simulink model "plcTest"  (R2018a)
settings: Solver=VariableStepAuto  StartTime=0.0  StopTime=5  RelTol=1e-3
values from neighbouring files (symbols this model uses):
  structureType = -1.0    [test.sldd]
undefined symbols (not defined in the file or in its folder): a_elem, b_elem, DB1
libraries: plcLibrary x1
settings Model: DataDictionary=test.sldd  Creator=thomas  LastModifiedBy=thomas

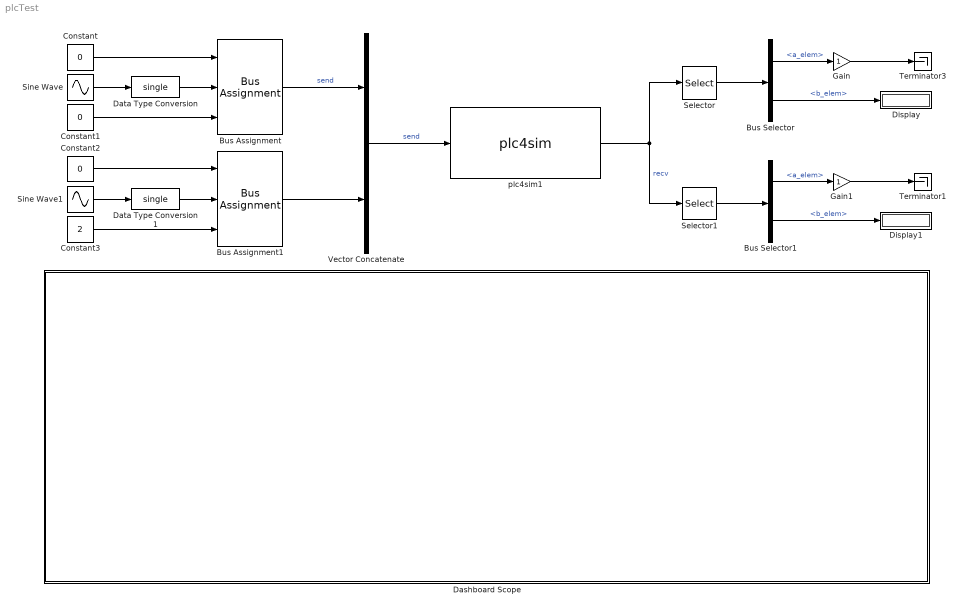
== system plcTest ==
  Bus Assignment : BusAssignment  AssignedSignals=a_elem,b_elem
  Bus Assignment1 : BusAssignment  AssignedSignals=a_elem,b_elem
  Bus Selector : BusSelector  OutputSignals=a_elem,b_elem
  Bus Selector1 : BusSelector  OutputSignals=a_elem,b_elem
  Constant : Constant  Value=0  OutDataTypeStr=Bus: structureType
  Constant1 : Constant  Value=0  OutDataTypeStr=uint8
  Constant2 : Constant  Value=0  OutDataTypeStr=Bus: structureType
  Constant3 : Constant  Value=2  OutDataTypeStr=uint8
  Dashboard Scope : Subsystem  DialogController=hmiCreateDDGDialog  IsWebBlock=on  mask(MWDashboardBlock){webBlockId=307e5b85-c1be-4a92-a345-0b0d646f5c8b, webBlockType=sdiscope, ShowInitialText=on, HMISrcModelName=plcTest}
      mask prompts: webBlockId "WebBlock Id"; webBlockType "WebBlock Type"; HMISrcModelName "Source Model"
      mask help: SimulinkHMI:dialogs:HMIScopeDialogDesc
      mask Help: helpview([docroot '/mapfiles/simulink.map'], 'hmi_scope')
      mask Display:
      | if strcmp(get_param(bdroot(gcb),'BlockDiagramType'), 'library')
      |     image([(matlabroot) '/toolbox/simulink/hmi/icons/DashboardScope.png']);
      | end
  Data Type Conversion : DataTypeConversion  OutDataTypeStr=single
  Data Type Conversion1 : DataTypeConversion  OutDataTypeStr=single
  Display : Display
  Display1 : Display
  Gain : Gain
  Gain1 : Gain
  Selector : Selector  InputPortWidth=2  IndexOptions=Index vector (dialog)  Indices=1  OutputSizes=1
  Selector1 : Selector  InputPortWidth=2  IndexOptions=Index vector (dialog)  Indices=2  OutputSizes=1
  Sine Wave : Sin  Bias=[1 -1]  Frequency=[2 5]  SampleTime=0.01
  Sine Wave1 : Sin  Bias=[1 -1]  Frequency=[7 9]  SampleTime=0.01
  Terminator1 : Terminator
  Terminator3 : Terminator
  Vector Concatenate : Concatenate
  plc4sim1 : plcLibrary/plc4sim  ts=0.05  nInputs=1  nOutputs=1  connStr=s7:tcp://0.0.0.0:102  writeStr=%DB1:8.0:structureType[1,2]  readStr=%DB1:8.0:structureType[1,2]  transport=TCP  protocol=S7  connItem1=0  connItem2=0  connItem3=0  ipTypeSelector=Inherit: auto  ip1_Type=structureType  ip1_Dims=1,2  ip1_Pos=%DB1:8.0  ip2_Type=0  ip2_Dims=0  ip2_Pos=0  ip3_Type=0  ip3_Dims=0  ip3_Pos=0  ip4_Type=double  ip4_Dims=1,1  ip4_Pos=%DB1:0.0  ip5_Type=double  ip5_Dims=1,1  ip5_Pos=%DB1:0.0  ip6_Type=double  ip6_Dims=1,1  ip6_Pos=%DB1:0.0  ip7_Type=double  ip7_Dims=1,1  ip7_Pos=%DB1:0.0  ip8_Type=double  ip8_Dims=1,1  ip8_Pos=%DB1:0.0  ip9_Type=double  ip9_Dims=1,1  ip9_Pos=%DB1:0.0  ip10_Type=double  ip10_Dims=1,1  ip10_Pos=%DB1:0.0  ip11_Type=double  ip11_Dims=1,1  ip11_Pos=%DB1:0.0  ip12_Type=double  ip12_Dims=1,1  ip12_Pos=%DB1:0.0  ip13_Type=double  ip13_Dims=1,1  ip13_Pos=%DB1:0.0  ip14_Type=double  ip14_Dims=1,1  ip14_Pos=%DB1:0.0  ip15_Type=double  ip15_Dims=1,1  ip15_Pos=%DB1:0.0  ip16_Type=double  ip16_Dims=1,1  ip16_Pos=%DB1:0.0  ip17_Type=double  ip17_Dims=1,1  ip17_Pos=%DB1:0.0  ip18_Type=double  ip18_Dims=1,1  ip18_Pos=%DB1:0.0  ip19_Type=double  ip19_Dims=1,1  ip19_Pos=%DB1:0.0  ip20_Type=double  ip20_Dims=1,1  ip20_Pos=%DB1:0.0  ip21_Type=double  ip21_Dims=1,1  ip21_Pos=%DB1:0.0  ip22_Type=double  ip22_Dims=1,1  ip22_Pos=%DB1:0.0  ip23_Type=double  ip23_Dims=1,1  ip23_Pos=%DB1:0.0  ip24_Type=double  ip24_Dims=1,1  ip24_Pos=%DB1:0.0  ip25_Type=double  ip25_Dims=1,1  ip25_Pos=%DB1:0.0  ip26_Type=double  ip26_Dims=1,1  ip26_Pos=%DB1:0.0  ip27_Type=double  ip27_Dims=1,1  ip27_Pos=%DB1:0.0  ip28_Type=double  ip28_Dims=1,1  ip28_Pos=%DB1:0.0  ip29_Type=double  ip29_Dims=1,1  ip29_Pos=%DB1:0.0  ip30_Type=double  ip30_Dims=1,1  ip30_Pos=%DB1:0.0  ip31_Type=double  ip31_Dims=1,1  ip31_Pos=%DB1:0.0  ip32_Type=double  ip32_Dims=1,1  ip32_Pos=%DB1:0.0  opTypeSelector=Inherit: auto  op1_Type=structureType  op1_Dims=1,2  op1_Pos=%DB1:8.0  op2_Type=0  op2_Dims=0  op2_Pos=0  op3_Type=0  op3_Dims=0  op3_Pos=0  op4_Type=double  op4_Dims=1,1  op4_Pos=%DB1:0.0  op5_Type=double  op5_Dims=1,1  op5_Pos=%DB1:0.0  op6_Type=double  op6_Dims=1,1  op6_Pos=%DB1:0.0  op7_Type=double  op7_Dims=1,1  op7_Pos=%DB1:0.0  op8_Type=double  op8_Dims=1,1  op8_Pos=%DB1:0.0  op9_Type=double  op9_Dims=1,1  op9_Pos=%DB1:0.0  op10_Type=double  op10_Dims=1,1  op10_Pos=%DB1:0.0  op11_Type=double  op11_Dims=1,1  op11_Pos=%DB1:0.0  op12_Type=double  op12_Dims=1,1  op12_Pos=%DB1:0.0  op13_Type=double  op13_Dims=1,1  op13_Pos=%DB1:0.0  op14_Type=double  op14_Dims=1,1  op14_Pos=%DB1:0.0  op15_Type=double  op15_Dims=1,1  op15_Pos=%DB1:0.0  op16_Type=double  op16_Dims=1,1  op16_Pos=%DB1:0.0  op17_Type=double  op17_Dims=1,1  op17_Pos=%DB1:0.0  op18_Type=double  op18_Dims=1,1  op18_Pos=%DB1:0.0  op19_Type=double  op19_Dims=1,1  op19_Pos=%DB1:0.0  op20_Type=double  op20_Dims=1,1  op20_Pos=%DB1:0.0  op21_Type=double  op21_Dims=1,1  op21_Pos=%DB1:0.0  op22_Type=double  op22_Dims=1,1  op22_Pos=%DB1:0.0  op23_Type=double  op23_Dims=1,1  op23_Pos=%DB1:0.0  op24_Type=double  op24_Dims=1,1  op24_Pos=%DB1:0.0  op25_Type=double  op25_Dims=1,1  op25_Pos=%DB1:0.0  op26_Type=double  op26_Dims=1,1  op26_Pos=%DB1:0.0  op27_Type=double  op27_Dims=1,1  op27_Pos=%DB1:0.0  op28_Type=double  op28_Dims=1,1  op28_Pos=%DB1:0.0  op29_Type=double  op29_Dims=1,1  op29_Pos=%DB1:0.0  op30_Type=double  op30_Dims=1,1  op30_Pos=%DB1:0.0  op31_Type=double  op31_Dims=1,1  op31_Pos=%DB1:0.0  op32_Type=double  op32_Dims=1,1  op32_Pos=%DB1:0.0  mask(plc4sim){}
  wires:
  Sine Wave/1 -> Data Type Conversion/1
  Data Type Conversion/1 -> Bus Assignment/2
  Bus Assignment/1 -> Vector Concatenate/1  "send"
  Constant/1 -> Bus Assignment/1
  plc4sim1/1 -> Selector/1, Selector1/1  "recv"
  Bus Selector/2 -> Display/1  "<b_elem>"
  Constant1/1 -> Bus Assignment/3
  Bus Selector/1 -> Gain/1  "<a_elem>"
  Gain/1 -> Terminator3/1
  Vector Concatenate/1 -> plc4sim1/1  "send"
  Selector/1 -> Bus Selector/1
  Constant3/1 -> Bus Assignment1/3
  Constant2/1 -> Bus Assignment1/1
  Data Type Conversion1/1 -> Bus Assignment1/2
  Sine Wave1/1 -> Data Type Conversion1/1
  Bus Assignment1/1 -> Vector Concatenate/2
  Selector1/1 -> Bus Selector1/1
  Gain1/1 -> Terminator1/1
  Bus Selector1/1 -> Gain1/1  "<a_elem>"
  Bus Selector1/2 -> Display1/1  "<b_elem>"

== system plcTest/Dashboard Scope ==
